simulink model "F_sim"  (R2017a)
settings: Solver=ode45  StartTime=0.0  StopTime=10000  MaxStep=.1  RelTol=1e-3  EnableMultiTasking=on
InitFcn:
  | addpath ./..
  | F_param
undefined symbols (not defined in the file): F_animation
libraries: simulink x3
settings Model: Creator=beard  LastModifiedBy=Mat Haskell
settings DataIOCC: LimitDataPoints=on  SaveFormat=Array  SignalLoggingSaveFormat=ModelDataLogs
settings OptimizationCC: ExpressionDepthLimit=2147483647  InitFltsAndDblsToZero=on  LifeSpan=inf
settings DebuggingCC: UnderspecifiedInitializationDetection=Classic  MergeDetectMultiDrivingBlocksExec=none  SolverPrmCheckMsg=warning  FcnCallInpInsideContextMsg=warning  StateNameClashWarn=warning  SFUnexpectedBacktrackingDiag=warning  SFNoUnconditionalDefaultTransitionDiag=warning  SFExecutionAtInitializationDiag=none
settings HardwareCC: ProdBitPerPointer=32  ProdBitPerSizeT=32  ProdBitPerPtrDiffT=32  ProdLargestAtomicFloat=None  ProdIntDivRoundTo=Undefined  ProdEndianess=Unspecified  ProdWordSize=32  ProdHWDeviceType=32-bit Generic
settings ModelReferenceCC: PropagateSignalLabelsOutOfModel=off
settings GRTTargetCC: TargetLangStandard=C89/C90 (ANSI)  GeneratePreprocessorConditionals=Disable all  CombineOutputUpdateFcns=off  GRTInterface=on
settings ConfigComp: CovMetricSettings=dw  CovHtmlReporting=on  CovSaveCumulativeToWorkspaceVar=on  CovSaveSingleToWorkspaceVar=on  CovExternalEMLEnable=off

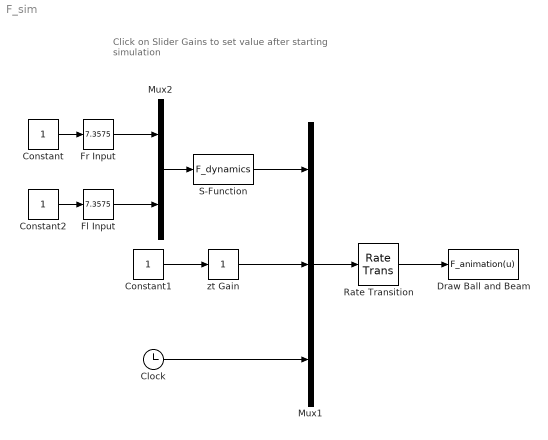
== system F_sim ==
  note: Click on Slider Gains to set value
      | after starting simulation
  Clock : Clock
  Constant : Constant
  Constant1 : Constant
  Constant2 : Constant
  Draw Ball and Beam : MATLABFcn  InitFcn=|  MATLABFcn=F_animation(u)  OutputDimensions=0
      | clear;clc
      | F_param
  Fl Input : simulink/Math Operations/Slider Gain  gain=7.3575  low=7.357  high=7.358
  Fr Input : simulink/Math Operations/Slider Gain  gain=7.3575  low=7  high=7.5
  Mux1 : Mux  Inputs=3
  Mux2 : Mux  Inputs=2
  Rate Transition : RateTransition  OutPortSampleTime=P.t_plot
  S-Function : S-Function  FunctionName=F_dynamics  Parameters=P  SFunctionDeploymentMode=off  EnableBusSupport=off
  zt Gain : simulink/Math Operations/Slider Gain  gain=1  low=0  high=5
  wires:
  Clock/1 -> Mux1/3
  Mux1/1 -> Rate Transition/1
  Rate Transition/1 -> Draw Ball and Beam/1
  S-Function/1 -> Mux1/1
  Constant/1 -> Fr Input/1
  zt Gain/1 -> Mux1/2
  Constant1/1 -> zt Gain/1
  Mux2/1 -> S-Function/1
  Fr Input/1 -> Mux2/1
  Fl Input/1 -> Mux2/2
  Constant2/1 -> Fl Input/1
